simulink model "ShuntingRes"  (R2022b)
settings: Solver=VariableStepAuto  StartTime=0.0  StopTime=1800  FixedStep=1e-3  RelTol=1e-3
undefined symbols (not defined in the file): Ion, Lithium
libraries: spsIdealSwitchLib x2, simulink x2, spsBatteryLib x1, spsParallelRLCBranchLib x1, spspowerguiLib x1
settings Model: Creator=MAAM  LastModifiedBy=MAAM
settings SolverCC: ZeroCrossAlgorithm=Adaptive
settings DebuggingCC: IgnoredZcDiagnostic=none  UnderSpecifiedDimensionMsg=warning

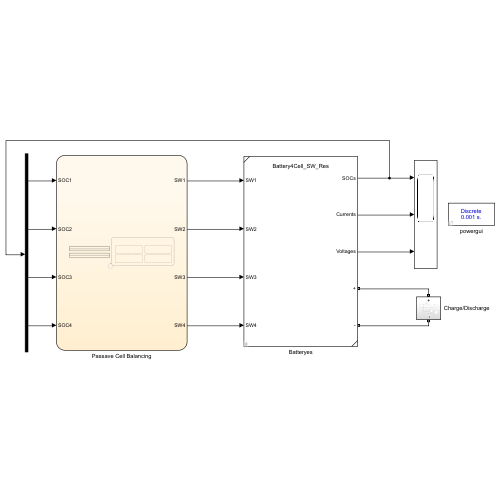
[thumbnail: Simulink's stored preview of the top-level diagram]
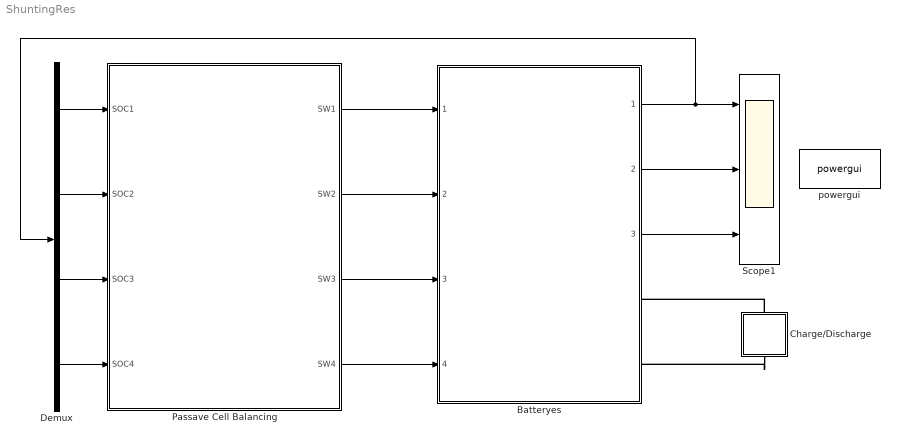
== system ShuntingRes ==
  Batteryes : Subsystem  ReferencedSubsystem=Battery4Cell_SW_Res  V0=3.7  Ah=5.20  SOC1=70  SOC2=50  SOC3=60  SOC4=85  R=0.25
  Charge/Discharge : Subsystem
  Demux : Demux
  Passave Cell Balancing : Stateflow chart  TreatAsAtomicUnit=on
  Scope1 : Scope  NumInputPorts=3
  powergui : spspowerguiLib/powergui  Priority=1  SimulationMode=Discrete  SampleTime=0.001  frequency=60  Iterations=50  frequencyindice=0  Pbase=100e6  ErrMax=1e-4  UnitsV=kV  UnitsW=MW  buscounter=0  FunctionMessages=off  echomessages=off  EnableUseOfTLC=off  CurrentSourceSwitches=off  DisableSnubberDevices=off  DisableRonSwitches=off  DisableVfSwitches=off  DisplayEquations=off  AutomaticDiscreteSolvers=off  SolverType=Tustin/Backward Euler (TBE)  Interpol=off  ExternalGateDelay=off  methode=off  Ts=100  x0status=blocks  SPID=on  SwTol=0  HookPort=off  NonlinearTolerance=1e-4  nMaxIteration=100  ContinueOnMaxIteration=off  RestoreLinks=warning  ResistiveCurrentMeasurement=off  Frange=[0:2:500]  Ylog=off  Xlog=on  ShowGrid=off  save=off  variable=ZData  structure=0  ZoomFFT=off  StartTime=0.0  cycles=1  DisplayStyle=1  fundamental=60  FreqAxis=off  MaxFrequency=1000  frequencyindicesteady=1  RmsSteady=1  display=off
  wires:
  Batteryes/1 -> Demux/1, Scope1/1
  Batteryes/3 -> Scope1/3
  Batteryes/2 -> Scope1/2
  Passave Cell Balancing/2(SW2) -> Batteryes/2
  Passave Cell Balancing/3(SW3) -> Batteryes/3
  Passave Cell Balancing/4(SW4) -> Batteryes/4
  Demux/1 -> Passave Cell Balancing/1(SOC1)
  Demux/2 -> Passave Cell Balancing/2(SOC2)
  Demux/3 -> Passave Cell Balancing/3(SOC3)
  Demux/4 -> Passave Cell Balancing/4(SOC4)
  Passave Cell Balancing/1(SW1) -> Batteryes/1
  connections:
  Charge/Discharge/LConn1 -- Batteryes/RConn1
  Charge/Discharge/RConn1 -- Batteryes/RConn2

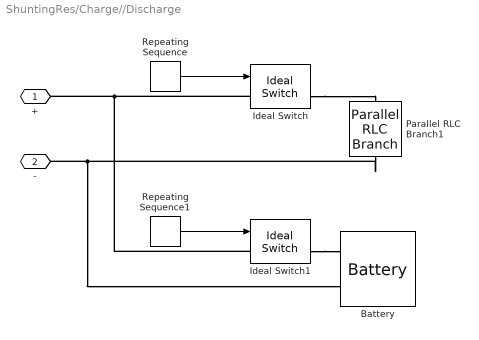
== system ShuntingRes/Charge//Discharge ==
  Battery : spsBatteryLib/Battery  BatType=Lithium-Ion  ShowTempParam=off  ThermalPreset=no  ShowAgeParam=off  NomV=15  NomQ=100  SOC=100  Batt_Tr=30  PresetModel=on  MaxQ=100  MinV=11.25  FullV=17.4598  Dis_rate=43.4783  R=0.0015  Normal_OP=90.4348  expZone="[16.2058      4.91304]"  current=[6.5 13 32.5]  Units=Time  Tci=20  NomT=20  T2=-30  MaxQ2=4.8  FullV2=7.1  Normal_OP2=5.655  expZone2="[6.58           1]"  Rca=0.6  ti=2000  Dp=0  Neq0=0  Tsim=1e6  Ta1=25  Qeol=5.4*0.9  Reol=0.013333*1.2  Char_age=[2.3478, 3]  Dis_age=[2.3478, 10]  N1=1500  N2=10500  N3=1000  N4=1400  Ta2=45  N5=950
  Ideal Switch : spsIdealSwitchLib/Ideal Switch  Ron=0.001  Lon=0  IC=0  Rs=1e5  Cs=inf  Measurements=on
  Ideal Switch1 : spsIdealSwitchLib/Ideal Switch  Ron=0.001  Lon=0  IC=0  Rs=1e5  Cs=inf  Measurements=on
  Parallel RLC Branch1 : spsParallelRLCBranchLib/Parallel RLC Branch  LConnTagsString=a  RConnTagsString=__new0  BranchType=R  Resistance=1  Inductance=1e-3  SetiL0=off  InitialCurrent=0  Capacitance=1e-6  Setx0=off  InitialVoltage=0  Measurements=None
  Repeating Sequence : simulink/Sources/Repeating Sequence  rep_seq_t=[0 600 600.001 1000 1000.001]  rep_seq_y=[0 0 1 1 0]
  Repeating Sequence1 : simulink/Sources/Repeating Sequence  rep_seq_t=[0 1000 1000.001 1800 1800.001]  rep_seq_y=[0 0 1 1 0]
  + : PMIOPort  Side=Left
  - : PMIOPort  Port=2  Side=Right
  wires:
  Repeating Sequence/1 -> Ideal Switch/1
  Repeating Sequence1/1 -> Ideal Switch1/1
  connections:
  Ideal Switch/RConn1 -- Parallel RLC Branch1/LConn1
  Parallel RLC Branch1/RConn1 -- Battery/LConn2 -- -/RConn1
  Ideal Switch/LConn1 -- Ideal Switch1/LConn1 -- +/RConn1
  Ideal Switch1/RConn1 -- Battery/LConn1

== stateflow chart ShuntingRes/Passave Cell Balancing ==
  state Super
    en:
    LowVolt = getLowSOC(SOC1, SOC2, SOC3, SOC4);
    state SW1_Out [parallel]
      en:
      SW1 = setSwOut(SOC1, LowVolt);
      settings: executionOrder=1
    state SW2_Out [parallel]
      en:
      SW2 = setSwOut(SOC2, LowVolt);
      settings: executionOrder=2
    state SW3_Out [parallel]
      en:
      SW3 = setSwOut(SOC3, LowVolt);
      settings: executionOrder=3
    state SW4_Out [parallel]
      en:
      SW4 = setSwOut(SOC4, LowVolt);
      settings: executionOrder=4
  state V_Low  = getLowSOC(In1, In2, In3, In4) [function]
    (default) -> (junction 2)
    (junction 2) -> (junction 21) [order 1] : [In1 <= In2]
    (junction 21) -> (junction 24) [order 1] : [In1 <= In3]
    (junction 24) -> (junction 26) [order 1] : [In1 <= In4]
    (junction 2) -> (junction 43) [order 2]
    (junction 21) -> (junction 62) [order 2]
    (junction 24) -> (junction 75) [order 2]
    (junction 26) -> (junction 27) : {V_Low = In1;}
    (junction 43) -> (junction 45) : [In2 <= In3]
    (junction 45) -> (junction 47) [order 1] : [In2 <= In4]
    (junction 45) -> (junction 29) [order 2]
    (junction 47) -> (junction 49) : {V_Low = In2;}
    (junction 62) -> (junction 31)
    (junction 31) -> (junction 61) [order 1] : [In3 <= In4]
    (junction 31) -> (junction 73) [order 2]
    (junction 61) -> (junction 39) : {V_Low = In3;}
    (junction 73) -> (junction 29)
    (junction 29) -> (junction 75)
    (junction 75) -> (junction 59)
    (junction 59) -> (junction 36) : {V_Low = In4;}
  state Sw = setSwOut(Curr, Low) [function]
    (default) -> (junction 81)
    (junction 81) -> (junction 86) [order 1] : [abs(Curr - Low) > threshold]
    (junction 81) -> (junction 90) [order 2] : {Sw = false;}
    (junction 86) -> (junction 88) : {Sw = true;}
    (junction 88) -> (junction 90)
    (junction 90) -> (junction 94)
  Super -> Super
  data: In1 function_input double size=1; In2 function_input double size=1; In3 function_input double size=1; In4 function_input double size=1; V_Low function_output double size=1; Curr function_input double; Low function_input double; Sw function_output double; threshold constant double =0.001; SOC1 input double size=1; SOC2 input double size=1; SOC3 input double size=1; SOC4 input double size=1; SW1 output size=1; SW2 output size=1; SW3 output size=1; SW4 output size=1; LowVolt local double
